simulink subsystem "FTC_Unknown"  (R2020b)
settings: Solver=VariableStepAuto  StartTime=0.0  StopTime=10.0  RelTol=1e-3
values from neighbouring files (symbols this model uses):
  B = [0.25   -1.4142/(4*l)     1.4142/(4*l)     1/(4*c) ... (first row only)    [H250_LOEUnknown_400HzParam.m]
  g = (9.8)    (= 9.8)    [H250_LOEKnown_400HzParam.m]    (also in H250_LOEUnknown_400HzParam.m; H333_LOEKnown_400HzParam.m)
  J = (diag([0.0056 0.0056 0.0104]))    [H250_LOEKnown_400HzParam.m]    (also in H250_LOEUnknown_400HzParam.m; H333_LOEKnown_400HzParam.m = (diag([0.012 0.0120 0.02])))
  m = (0.752)    (= 0.752)    [H250_LOEKnown_400HzParam.m]    (also in H250_LOEUnknown_400HzParam.m; H333_LOEKnown_400HzParam.m = 1.13)
  M = ([ 1          1          1         1 ... (first row only)    [H250_LOEKnown_400HzParam.m]    (also in H250_LOEUnknown_400HzParam.m; H333_LOEKnown_400HzParam.m)
  MY_ATT_P = Pixhawk_CSC.Parameter( {single(8), 'MY_ATT_P'}  )    [H250_LOEKnown_400HzParam.m]    (also in H250_LOEUnknown_400HzParam.m = Pixhawk_CSC.Parameter( {single(3), 'MY_ATT_P'}  ); H333_LOEKnown_400HzParam.m)
  MY_ATT_P_YAW = Pixhawk_CSC.Parameter( {single(0), 'MY_ATT_P_YAW'}  )    [H250_LOEKnown_400HzParam.m]    (also in H250_LOEUnknown_400HzParam.m = Pixhawk_CSC.Parameter( {single(0.0), 'MY_ATT_P_YAW'}  ); H333_LOEKnown_400HzParam.m)
  MY_POS_P = Pixhawk_CSC.Parameter( {single(0.5), 'MY_POS_P'}  )    [H250_LOEKnown_400HzParam.m]    (also in H250_LOEUnknown_400HzParam.m; H333_LOEKnown_400HzParam.m)
  MY_RATE_P = Pixhawk_CSC.Parameter( {single(12), 'MY_RATE_P'}  )    [H250_LOEKnown_400HzParam.m]    (also in H250_LOEUnknown_400HzParam.m = Pixhawk_CSC.Parameter( {single(14), 'MY_RATE_P'}  ); H333_LOEKnown_400HzParam.m)
  MY_RATE_P_YAW = Pixhawk_CSC.Parameter( {single(0.3), 'MY_RATE_P_YAW'}  )    [H250_LOEKnown_400HzParam.m]    (also in H250_LOEUnknown_400HzParam.m = Pixhawk_CSC.Parameter( {single(0.0), 'MY_RATE_P_YAW'}  ); H333_LOEKnown_400HzParam.m)
  MY_SAT_AD = Pixhawk_CSC.Parameter({single(0.13), 'MY_SAT_AD'} )    [H250_LOEKnown_400HzParam.m]    (also in H250_LOEUnknown_400HzParam.m; H333_LOEKnown_400HzParam.m)
  MY_TAU_P_A = Pixhawk_CSC.Parameter( {single(0), 'MY_TAU_P_A'}  )    [H250_LOEKnown_400HzParam.m]    (also in H250_LOEUnknown_400HzParam.m = Pixhawk_CSC.Parameter( {single(0.0), 'MY_TAU_P_A'}  ); H333_LOEKnown_400HzParam.m)
  MY_TAU_P_A_YAW = Pixhawk_CSC.Parameter( {single(0), 'MY_TAU_P_A_YAW'}  )    [H250_LOEKnown_400HzParam.m]    (also in H250_LOEUnknown_400HzParam.m; H333_LOEKnown_400HzParam.m)
  MY_TAU_P_P = Pixhawk_CSC.Parameter( {single(1.5), 'MY_TAU_P_P'}  )    [H250_LOEKnown_400HzParam.m]    (also in H250_LOEUnknown_400HzParam.m = Pixhawk_CSC.Parameter( {single(1.3), 'MY_TAU_P_P'}  ); H333_LOEKnown_400HzParam.m)
  MY_TAU_P_P_YAW = Pixhawk_CSC.Parameter( {single(0.1), 'MY_TAU_P_P_YAW'}  )    [H250_LOEKnown_400HzParam.m]    (also in H250_LOEUnknown_400HzParam.m; H333_LOEKnown_400HzParam.m)
  MY_VEL_P = Pixhawk_CSC.Parameter( {single(0.8), 'MY_VEL_P'}  )    [H250_LOEKnown_400HzParam.m]    (also in H250_LOEUnknown_400HzParam.m; H333_LOEKnown_400HzParam.m)
  T00 = single([m*g/4 m*g/4 m*g/4 m*g/4]')    [H250_LOEKnown_400HzParam.m]    (also in H250_LOEUnknown_400HzParam.m; H333_LOEKnown_400HzParam.m)
  Tf = 0.06    [H250_LOEKnown_400HzParam.m]    (also in H250_LOEUnknown_400HzParam.m; H333_LOEKnown_400HzParam.m)
  Tmotorbar = (0.035)    (= 0.035)    [H250_LOEKnown_400HzParam.m]    (also in H250_LOEUnknown_400HzParam.m = 0.032; H333_LOEKnown_400HzParam.m)
  Ts = 1/400    (= 0.0025)    [H250_LOEKnown_400HzParam.m]    (also in H250_LOEUnknown_400HzParam.m; H333_LOEKnown_400HzParam.m)
libraries: discretizing x10, simulink x1, sharedtransform x1, pid_lib x1, pixhawk_slib_uORB_RW x1
settings Model: Creator=kcx06  LastModifiedBy=kcx06

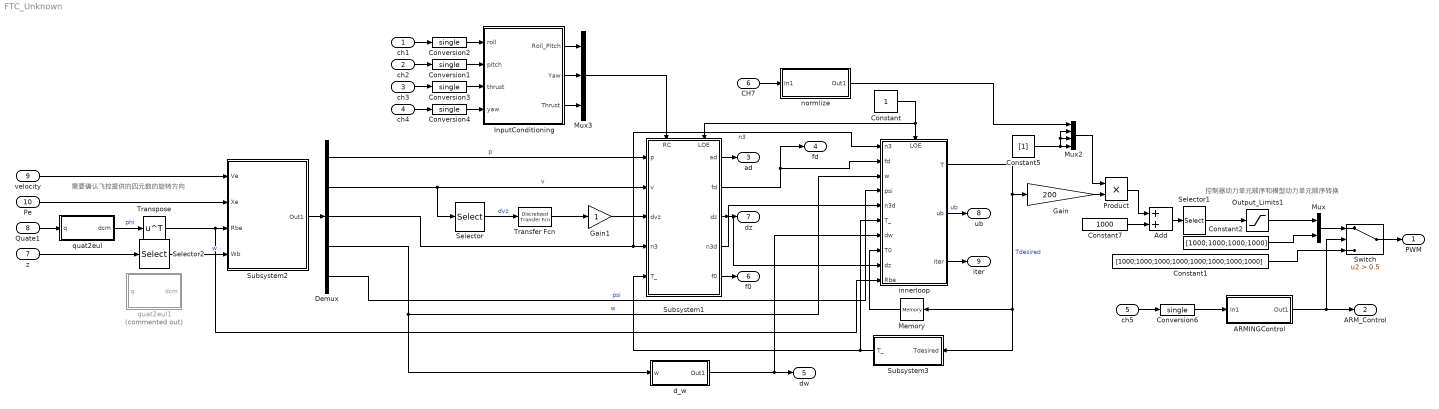
== system FTC_Unknown ==
  note: 需要确认飞控提供的四元数的旋转方向
  note: 控制器动力单元顺序和模型动力单元顺序转换
  ch1 : Inport  OutDataTypeStr=uint16  PortDimensions=1
  ch2 : Inport  Port=2  OutDataTypeStr=uint16  PortDimensions=1
  ch3 : Inport  Port=3  OutDataTypeStr=uint16  PortDimensions=1
  ch4 : Inport  Port=4  OutDataTypeStr=uint16  PortDimensions=1
  ch5 : Inport  Port=5  OutDataTypeStr=uint16  PortDimensions=1  Interpolate=off
  CH7 : Inport  Port=6
  z : Inport  Port=7
  Quate1 : Inport  Port=8
  velocity : Inport  Port=9
  Pe : Inport  Port=10
  ARMINGControl : Subsystem
  Add : Sum
  Constant : Constant  OutDataTypeStr=single
  Constant1 : Constant  Value=[1000;1000;1000;1000;1000;1000;1000;1000]  OutDataTypeStr=single
  Constant2 : Constant  Value=[1000;1000;1000;1000]  OutDataTypeStr=single
  Constant5 : Constant  Value=[1]  OutDataTypeStr=single
  Constant7 : Constant  Value=1000  OutDataTypeStr=single
  Conversion{1..4,6} (5 alike) : DataTypeConversion  OutDataTypeStr=single
  Demux : Demux  Outputs=[3 3 3 3 1]
  Gain : Gain  Gain=200
  Gain1 : Gain
  InputConditioning : Subsystem
  Memory : Memory  InitialCondition=T00
  Mux : Mux  Inputs=2
  Mux2 : Mux
  Mux3 : Mux  Inputs=3
  Output_Limits1 : Saturate  UpperLimit=2000  LowerLimit=1000
  Product : Product
  Selector : Selector  IndexMode=Zero-based  InputPortWidth=3  IndexOptions=Index vector (dialog)  Indices=[2]  OutputSizes=1
  Selector1 : Selector  IndexMode=Zero-based  InputPortWidth=4  IndexOptions=Index vector (dialog)  Indices=[0 2 3 1]  OutputSizes=1
  Selector2 : Selector  IndexMode=Zero-based  InputPortWidth=3  IndexOptions=Index vector (dialog)  Indices=[0 1 2]  OutputSizes=1
  Subsystem1 : Subsystem
      settings: PortSchema="{\"entries\":[{\"content\":{\"sides\":[{\"content\":{\"connectorIds\":[\"In1\",\"In2\",\"In3\",\"In4\",\"In5\"]},\"type\":\"ConnectorPlacement.EquallySpacedRectSide\",\"uuid\":\"59983f3e-2daf-41bd-bc3f-074c85f4b2eb\"},{\"content\":{\"connectorIds\":[\"Out1\",\"Out2\",\"Out3\",\"Out4\",\"Out5\"],\"side\":\"RIGHT\"},\"type\":\"ConnectorPlacement.EquallySpacedRectSide\",\"uuid\":\"6ee11e40-7870-4737-b9e6-fd7c25119100\"},{\"content\":{\"connectorIds\":[\"In6\",\"In7\"],\"side\":\"TOP\"},\"type\":\"ConnectorPlacement.EquallySpacedRectSide\",\"uuid\":\"847e9a02-4621-4cf8-a675-1479afa28be0\"}]},\"type\":\"ConnectorPlacement.EquallySpacedConnector\",\"uuid\":\"28981c41-e87e-4da3-ac2d-04a56d75ff2b\"}],\"packageUris\":[\"http://schema.mathworks.com/mf0/Connector/19700101\"],\"version\":\"1.0\"}"
  Subsystem2 : Subsystem
  Subsystem3 : Subsystem
  Switch : Switch  Criteria=u2 > Threshold  Threshold=0.5
  Transfer Fcn : discretizing/Discretized Transfer Fcn  Numerator=[1 0]  Denominator=[Tf 1]  AbsTol=auto  SampleTime=Ts  method=zoh  Wc=1
      settings: SourceProductBaseCode=SL
  Transpose : Math  Operator=transpose  SaturateOnIntegerOverflow=on
  d_w : Subsystem
  innerloop : Subsystem
      settings: PortSchema="{\"entries\":[{\"content\":{\"sides\":[{\"content\":{\"connectorIds\":[\"In1\",\"In2\",\"In3\",\"In4\",\"In5\",\"In6\",\"In7\",\"In8\",\"In9\",\"In10\"]},\"type\":\"ConnectorPlacement.EquallySpacedRectSide\",\"uuid\":\"43c6e1bd-c98b-47b4-98da-f51fdffff433\"},{\"content\":{\"connectorIds\":[\"Out1\",\"Out2\",\"Out3\"],\"side\":\"RIGHT\"},\"type\":\"ConnectorPlacement.EquallySpacedRectSide\",\"uuid\":\"ac1c9532-9168-4bf4-8fed-08d3fdc16453\"},{\"content\":{\"connectorIds\":[\"In11\"],\"side\":\"TOP\"},\"type\":\"ConnectorPlacement.EquallySpacedRectSide\",\"uuid\":\"32774b13-030c-47c6-b846-fc6c0ce2dd6f\"}]},\"type\":\"ConnectorPlacement.EquallySpacedConnector\",\"uuid\":\"dd62421a-d766-429a-a161-5a0f77c5a7ba\"}],\"packageUris\":[\"http://schema.mathworks.com/mf0/Connector/19700101\"],\"version\":\"1.0\"}"
  normlize : Subsystem
  quat2eul : MATLAB Function  TreatAsAtomicUnit=on
  quat2eul1 : MATLAB Function  Commented=on  TreatAsAtomicUnit=on
  PWM : Outport  PortDimensions=8  VectorParamsAs1DForOutWhenUnconnected=off
  ARM_Control : Outport  Port=2  PortDimensions=1  VectorParamsAs1DForOutWhenUnconnected=off
  ad : Outport  Port=3
  fd : Outport  Port=4
  dw : Outport  Port=5
  f0 : Outport  Port=6
  dz : Outport  Port=7
  ub : Outport  Port=8
  iter : Outport  Port=9
  wires:
  CH7/1 -> normlize/1(In1)
  z/1 -> Selector2/1
  Add/1 -> Selector1/1
  Subsystem1/1(ad) -> ad/1
  InputConditioning/3(Thrust) -> Mux3/3
  velocity/1 -> Subsystem2/1(Ve)
  Conversion2/1 -> InputConditioning/1(roll)
  Transpose/1 -> Subsystem2/3(Rbe), innerloop/10(Rbe)
  Demux/3 -> Subsystem1/4(n3), innerloop/1(n3)  "n3"
  InputConditioning/1(Roll_Pitch) -> Mux3/1
  Selector/1 -> Transfer Fcn/1  "dvz"
  Subsystem1/3(dz) -> dz/1, innerloop/9(dz)
  Product/1 -> Add/1
  Constant/1 -> innerloop/11(LOE), Subsystem1/7(LOE)
  Constant1/1 -> Switch/3
  Subsystem3/1(T_) -> Subsystem1/5(T_), innerloop/6(T_)
  quat2eul/1(dcm) -> Transpose/1  "phi"
  Demux/1 -> Subsystem1/1(p)  "p"
  Selector2/1 -> Subsystem2/4(Wb)  "w"
  innerloop/3(iter) -> iter/1
  Conversion3/1 -> InputConditioning/3(thrust)
  Pe/1 -> Subsystem2/2(Xe)
  ch5/1 -> Conversion6/1
  d_w/1(Out1) -> dw/1, innerloop/7(dw)
  Quate1/1 -> quat2eul/1(q)
  Demux/2 -> Subsystem1/2(v), Selector/1  "v"
  ch4/1 -> Conversion4/1
  Output_Limits1/1 -> Mux/1
  Constant7/1 -> Add/2
  Gain/1 -> Product/2
  Demux/4 -> innerloop/3(w), d_w/1(w)  "w"
  Subsystem1/2(fd) -> innerloop/2(fd), fd/1
  Memory/1 -> innerloop/8(T0)
  Demux/5 -> innerloop/4(psi)  "psi"
  ch1/1 -> Conversion2/1
  InputConditioning/2(Yaw) -> Mux3/2
  Selector1/1 -> Output_Limits1/1
  Transfer Fcn/1 -> Gain1/1
  innerloop/1(T) -> Gain/1, Memory/1, Subsystem3/1(Tdesired)  "Tdesired"
  ch2/1 -> Conversion1/1
  Conversion4/1 -> InputConditioning/4(yaw)
  normlize/1(Out1) -> Mux2/1
  Mux2/1 -> Product/1
  Mux/1 -> Switch/1
  Subsystem2/1(Out1) -> Demux/1
  innerloop/2(ub) -> ub/1  "ub"
  Conversion6/1 -> ARMINGControl/1(In1)
  Constant5/1 -> Mux2/4, Mux2/2, Mux2/3
  Switch/1 -> PWM/1
  Gain1/1 -> Subsystem1/3(dvz)
  ch3/1 -> Conversion3/1
  ARMINGControl/1(Out1) -> ARM_Control/1, Switch/2
  Subsystem1/5(f0) -> f0/1
  Mux3/1 -> Subsystem1/6(RC)
  Constant2/1 -> Mux/2
  Conversion1/1 -> InputConditioning/2(pitch)
  Subsystem1/4(n3d) -> innerloop/5(n3d)

== system FTC_Unknown/ARMINGControl ==
  In1 : Inport
  Compare To Constant3 : simulink/Logic and Bit Operations/Compare To Constant  relop=>=  const=uint16(1500)  OutDataTypeStr=boolean
  Out1 : Outport  VectorParamsAs1DForOutWhenUnconnected=off
  wires:
  In1/1 -> Compare To Constant3/1
  Compare To Constant3/1 -> Out1/1

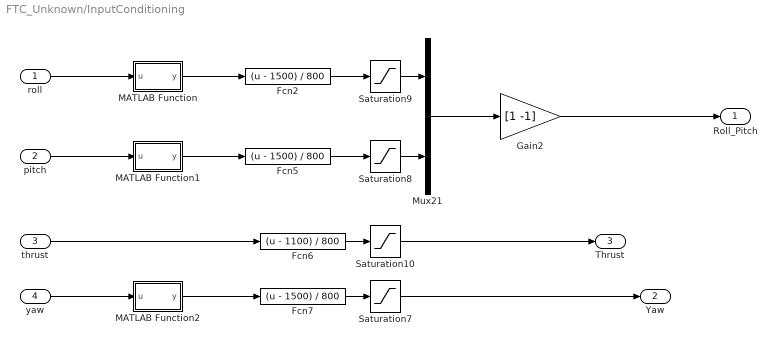
== system FTC_Unknown/InputConditioning ==
  roll : Inport
  pitch : Inport  Port=2
  thrust : Inport  Port=3
  yaw : Inport  Port=4
  Fcn2 : Fcn  Expr=(u - 1500) / 800
  Fcn5 : Fcn  Expr=(u - 1500) / 800
  Fcn6 : Fcn  Expr=(u - 1100) / 800
  Fcn7 : Fcn  Expr=(u - 1500) / 800
  Gain2 : Gain  Gain=[1 -1]  OutDataTypeStr=Inherit: Inherit via back propagation
  MATLAB Function : MATLAB Function  TreatAsAtomicUnit=on
  MATLAB Function1 : MATLAB Function  TreatAsAtomicUnit=on
  MATLAB Function2 : MATLAB Function  TreatAsAtomicUnit=on
  Mux21 : Mux  Inputs=2
  Saturation10 : Saturate  UpperLimit=1  LowerLimit=0
  Saturation7 : Saturate  UpperLimit=1  LowerLimit=-1
  Saturation8 : Saturate  UpperLimit=1  LowerLimit=-1
  Saturation9 : Saturate  UpperLimit=1  LowerLimit=-1
  Roll_Pitch : Outport  VectorParamsAs1DForOutWhenUnconnected=off
  Yaw : Outport  Port=2  VectorParamsAs1DForOutWhenUnconnected=off
  Thrust : Outport  Port=3  VectorParamsAs1DForOutWhenUnconnected=off
  wires:
  yaw/1 -> MATLAB Function2/1(u)
  MATLAB Function/1(y) -> Fcn2/1
  MATLAB Function1/1(y) -> Fcn5/1
  roll/1 -> MATLAB Function/1(u)
  thrust/1 -> Fcn6/1
  MATLAB Function2/1(y) -> Fcn7/1
  pitch/1 -> MATLAB Function1/1(u)
  Fcn7/1 -> Saturation7/1
  Saturation9/1 -> Mux21/1
  Fcn5/1 -> Saturation8/1
  Fcn2/1 -> Saturation9/1
  Fcn6/1 -> Saturation10/1
  Saturation8/1 -> Mux21/2
  Mux21/1 -> Gain2/1
  Gain2/1 -> Roll_Pitch/1
  Saturation7/1 -> Yaw/1
  Saturation10/1 -> Thrust/1

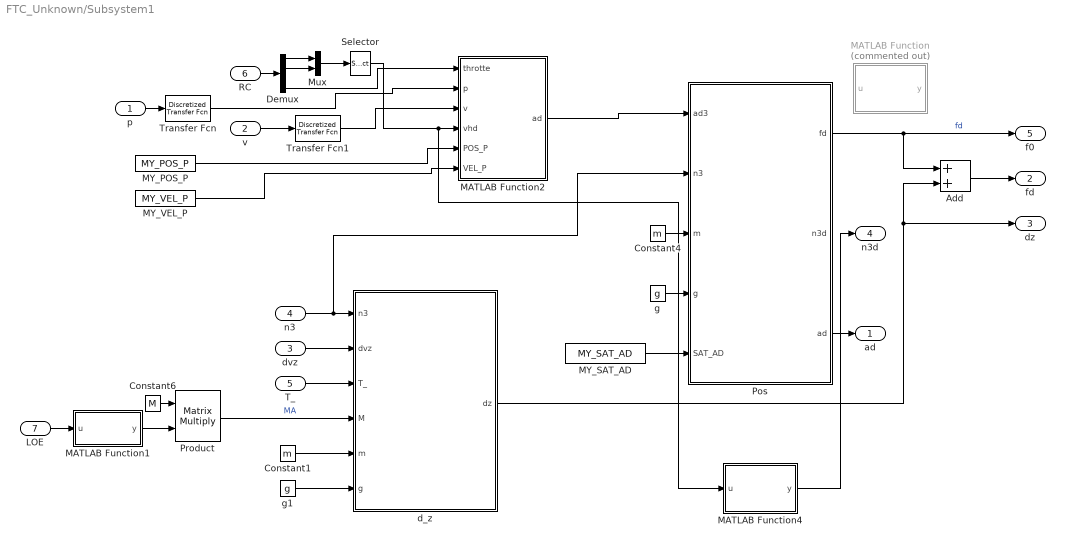
== system FTC_Unknown/Subsystem1 ==
  p : Inport
  v : Inport  Port=2
  dvz : Inport  Port=3
  n3 : Inport  Port=4
  T_ : Inport  Port=5
  RC : Inport  Port=6
  LOE : Inport  Port=7
  Add : Sum
  Constant1 : Constant  Value=m  OutDataTypeStr=single
  Constant4 : Constant  Value=m  OutDataTypeStr=single
  Constant6 : Constant  Value=M  OutDataTypeStr=single
  Demux : Demux
  MATLAB Function : MATLAB Function  Commented=on  TreatAsAtomicUnit=on
  MATLAB Function1 : MATLAB Function  TreatAsAtomicUnit=on
  MATLAB Function2 : MATLAB Function  TreatAsAtomicUnit=on
  MATLAB Function4 : MATLAB Function  TreatAsAtomicUnit=on
  MY_POS_P : Constant  Value=MY_POS_P
  MY_SAT_AD : Constant  Value=MY_SAT_AD
      settings: AttributesFormatString=|
      | 0.13
      | Default
  MY_VEL_P : Constant  Value=MY_VEL_P
  Mux : Mux  Inputs=2
  Pos : MATLAB Function  TreatAsAtomicUnit=on
  Product : Product  Multiplication=Matrix(*)
  Selector : Selector  IndexMode=Zero-based  InputPortWidth=2  IndexOptions=Index vector (dialog)  Indices=[1 0]  OutputSizes=1
  Transfer Fcn : discretizing/Discretized Transfer Fcn  Numerator=[1 ]  Denominator=[Tf 1]  AbsTol=auto  SampleTime=Ts  method=zoh  Wc=1
      settings: SourceProductBaseCode=SL
  Transfer Fcn1 : discretizing/Discretized Transfer Fcn  Numerator=[1 ]  Denominator=[Tf 1]  AbsTol=auto  SampleTime=Ts  method=zoh  Wc=1
      settings: SourceProductBaseCode=SL
  d_z : MATLAB Function  TreatAsAtomicUnit=on
  g : Constant  Value=g  OutDataTypeStr=single
  g1 : Constant  Value=g  OutDataTypeStr=single
  ad : Outport
  fd : Outport  Port=2
  dz : Outport  Port=3
  n3d : Outport  Port=4
  f0 : Outport  Port=5
  wires:
  MATLAB Function4/1(y) -> n3d/1
  MY_SAT_AD/1 -> Pos/5(SAT_AD)
  MY_VEL_P/1 -> MATLAB Function2/6(VEL_P)
  MY_POS_P/1 -> MATLAB Function2/5(POS_P)
  Selector/1 -> MATLAB Function2/4(vhd), MATLAB Function4/1(u)
  Mux/1 -> Selector/1
  Demux/2 -> Mux/2
  Demux/1 -> Mux/1
  Transfer Fcn1/1 -> MATLAB Function2/3(v)
  MATLAB Function2/1(ad) -> Pos/1(ad3)
  Demux/4 -> MATLAB Function2/1(throtte)
  RC/1 -> Demux/1
  Product/1 -> d_z/4(M)  "MA"
  Constant6/1 -> Product/1
  LOE/1 -> MATLAB Function1/1(u)
  MATLAB Function1/1(y) -> Product/2
  n3/1 -> d_z/1(n3), Pos/2(n3)
  Transfer Fcn/1 -> MATLAB Function2/2(p)
  d_z/1(dz) -> Add/2, dz/1
  Add/1 -> fd/1
  g1/1 -> d_z/6(g)
  Constant1/1 -> d_z/5(m)
  g/1 -> Pos/4(g)
  Constant4/1 -> Pos/3(m)
  v/1 -> Transfer Fcn1/1
  T_/1 -> d_z/3(T_)
  p/1 -> Transfer Fcn/1
  Pos/1(fd) -> Add/1, f0/1  "fd"
  dvz/1 -> d_z/2(dvz)
  Pos/3(ad) -> ad/1

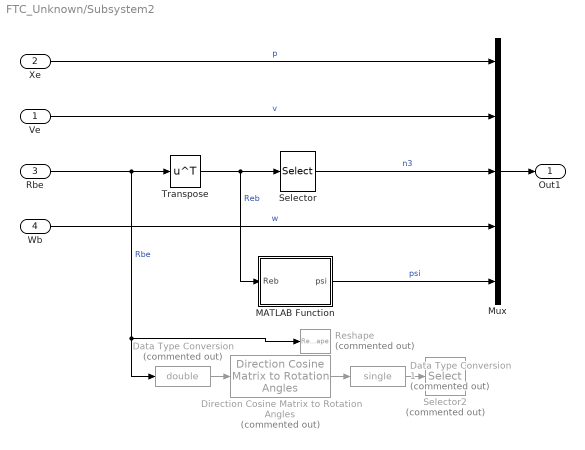
== system FTC_Unknown/Subsystem2 ==
  Ve : Inport
  Xe : Inport  Port=2
  Rbe : Inport  Port=3
  Wb : Inport  Port=4
  Data Type Conversion : DataTypeConversion  Commented=on  OutDataTypeStr=double
  Data Type Conversion1 : DataTypeConversion  Commented=on  OutDataTypeStr=single
  Direction Cosine Matrix to Rotation Angles : sharedtransform/Direction Cosine Matrix to Rotation Angles  Commented=on  rotationOrder=ZYX  aMode=aMode  action=None  tolerance=eps(2)
      settings: SourceProductBaseCode=AE,PW,MT,UV,VE,VP
  MATLAB Function : MATLAB Function  TreatAsAtomicUnit=on
  Mux : Mux  Inputs=[3 3 3 3 1]
  Reshape : Reshape  Commented=on
  Selector : Selector  NumberOfDimensions=2  IndexMode=Zero-based  InputPortWidth=3  IndexOptions=Select all,Index vector (dialog)  Indices=[1 3],2  OutputSizes=1,1
  Selector2 : Selector  Commented=on  InputPortWidth=3  IndexOptions=Index vector (dialog)  Indices=[3 2 1]  OutputSizes=1
  Transpose : Math  Operator=transpose  SaturateOnIntegerOverflow=on
  Out1 : Outport
  wires:
  Data Type Conversion1/1 -> Selector2/1
  Data Type Conversion/1 -> Direction Cosine Matrix to Rotation Angles/1
  Direction Cosine Matrix to Rotation Angles/1 -> Data Type Conversion1/1
  MATLAB Function/1(psi) -> Mux/5  "psi"
  Wb/1 -> Mux/4  "w"
  Mux/1 -> Out1/1
  Selector/1 -> Mux/3  "n3"
  Transpose/1 -> Selector/1, MATLAB Function/1(Reb)  "Reb"
  Rbe/1 -> Transpose/1, Data Type Conversion/1, Reshape/1  "Rbe"
  Ve/1 -> Mux/2  "v"
  Xe/1 -> Mux/1  "p"

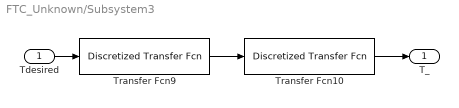
== system FTC_Unknown/Subsystem3 ==
  Tdesired : Inport
  Transfer Fcn10 : discretizing/Discretized Transfer Fcn  Numerator=[1]  Denominator=[Tmotorbar 1]  AbsTol=auto  SampleTime=Ts  method=zoh  Wc=1
      settings: SourceProductBaseCode=SL
  Transfer Fcn9 : discretizing/Discretized Transfer Fcn  Numerator=[1]  Denominator=[Tf 1]  AbsTol=auto  SampleTime=Ts  method=zoh  Wc=1
      settings: SourceProductBaseCode=SL
  T_ : Outport
  wires:
  Transfer Fcn9/1 -> Transfer Fcn10/1
  Tdesired/1 -> Transfer Fcn9/1
  Transfer Fcn10/1 -> T_/1

== system FTC_Unknown/d_w ==
  w : Inport
  Transfer Fcn4 : discretizing/Discretized Transfer Fcn  Numerator=[1 0]  Denominator=[Tf 1]  AbsTol=auto  SampleTime=Ts  method=zoh  Wc=1
      settings: SourceProductBaseCode=SL
  Out1 : Outport
  wires:
  Transfer Fcn4/1 -> Out1/1
  w/1 -> Transfer Fcn4/1

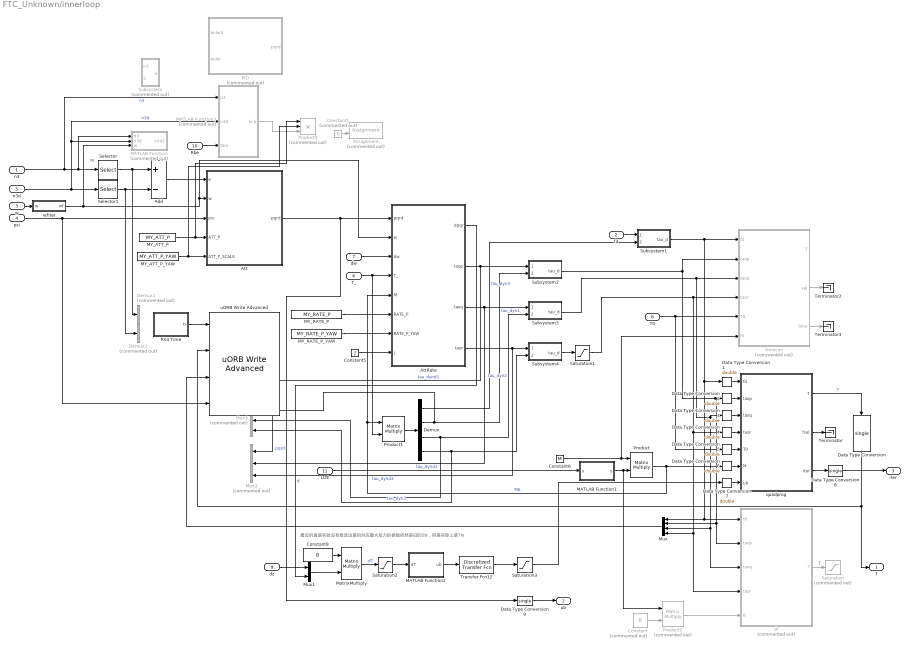
== system FTC_Unknown/innerloop ==
  note: 最近的真是实验没有修改这里的对应最大拉力的参数依然是旧的5N，但是实际上是7N
  note: PI
  n3 : Inport
  fd : Inport  Port=2
  w : Inport  Port=3
  psi : Inport  Port=4
  n3d : Inport  Port=5
  T_ : Inport  Port=6
  dw : Inport  Port=7
  T0 : Inport  Port=8
  dz : Inport  Port=9
  Rbe : Inport  Port=10
  LOE : Inport  Port=11
  Add : Sum  Inputs=+-
  Assignment : Assignment  Commented=on  DiagnosticForDimensions=Warning  IndexOptions=Index vector (dialog)  Indices=3  OutputSizes=1
  Att : MATLAB Function  TreatAsAtomicUnit=on
  AttRate : MATLAB Function  TreatAsAtomicUnit=on
  Constant : Constant  Commented=on  Value=B  OutDataTypeStr=single
  Constant1 : Constant  Commented=on  Value=0  OutDataTypeStr=single
  Constant5 : Constant  Value=J  OutDataTypeStr=single
  Constant6 : Constant  Value=M  OutDataTypeStr=single
  Constant8 : Constant  Value=B
  Data Type Conversion : DataTypeConversion  OutDataTypeStr=single
  Data Type Conversion{1..7} (7 alike) : DataTypeConversion  OutDataTypeStr=double
  Data Type Conversion8 : DataTypeConversion  OutDataTypeStr=single
  Data Type Conversion9 : DataTypeConversion  OutDataTypeStr=single
  Demux : Demux
  Demux1 : Demux  Commented=on  Outputs=2
  Demux2 : Demux  Commented=on  Outputs=2
  MATLAB Function : MATLAB Function  Commented=on  TreatAsAtomicUnit=on
  MATLAB Function1 : MATLAB Function  TreatAsAtomicUnit=on
  MATLAB Function2 : MATLAB Function  TreatAsAtomicUnit=on
  MATLAB Function3 : MATLAB Function  Commented=on  TreatAsAtomicUnit=on
  MY_ATT_P : Constant  Value=MY_ATT_P
  MY_ATT_P_YAW : Constant  Value=MY_ATT_P_YAW
  MY_RATE_P : Constant  Value=MY_RATE_P
  MY_RATE_P_YAW : Constant  Value=MY_RATE_P_YAW
  MatrixMultiply : Product  Multiplication=Matrix(*)
  Mux : Mux
  Mux1 : Mux  Inputs=2
  Mux2 : Mux  Commented=on  Inputs=3
  Mux3 : Mux  Commented=on  Inputs=3
  PID : MATLAB Function  Commented=on  TreatAsAtomicUnit=on
  PX4 Time : MATLAB Function  TreatAsAtomicUnit=on
  Product : Product  Multiplication=Matrix(*)
  Product1 : Product  Multiplication=Matrix(*)
  Product2 : Product  Commented=on  Multiplication=Matrix(*)
  Product3 : Product  Commented=on  Inputs=3
  Saturation : Saturate  Commented=on  UpperLimit=[3 3 3 3]  LowerLimit=[0 0 0 0]  OutDataTypeStr=single
  Saturation1 : Saturate  UpperLimit=0.075  LowerLimit=-0.075
  Saturation2 : Saturate  UpperLimit=5  LowerLimit=-5
  Saturation3 : Saturate  UpperLimit=5  LowerLimit=0
  Selector : Selector  IndexMode=Zero-based  InputPortWidth=3  IndexOptions=Index vector (dialog)  Indices=[0 1]  OutputSizes=1
  Selector1 : Selector  IndexMode=Zero-based  InputPortWidth=3  IndexOptions=Index vector (dialog)  Indices=[0 1]  OutputSizes=1
  Subsystem : Subsystem  Commented=on
  Subsystem1 : Subsystem
  Subsystem2 : Subsystem
  Subsystem3 : Subsystem
  Subsystem4 : Subsystem
  Terminator : Terminator
  Terminator2 : Terminator
  Terminator3 : Terminator
  Transfer Fcn12 : discretizing/Discretized Transfer Fcn  Numerator=[1]  Denominator="[1.7  1]"  AbsTol=auto  SampleTime=Ts  method=zoh  Wc=40
      link override Discrete Transfer Fcn: InitialStates=[5;5;5;5]
      settings: SourceProductBaseCode=SL
  dr : MATLAB Function  Commented=on  TreatAsAtomicUnit=on
  fmincon : MATLAB Function  Commented=on  TreatAsAtomicUnit=on
  quadprog : MATLAB Function  TreatAsAtomicUnit=on
  uORB Write Advanced : pixhawk_slib_uORB_RW/uORB Write Advanced  Ts=0  uORB_AdvtQueue=on  uORB_FieldEnabledArr="0  0  0  1  0  0  0  0  0  0  0"  uORB_Topic_str=0  uORB_Struct_DT="[1  1  1  1  1]"  BlockInputCount=5  uORB_StructParams="[\"voltage_v\",\"voltage_filtered_v\",\"current_a\",\"current_filtered_a\",\"remaining\"]"  uORB_PortSizes="[1  1  1  1]"  MsgSizeOf=0  MW_update=true
      settings: SourceProductName=Pixhawk Target Blocks
  wfiter : Subsystem
  T : Outport  PortDimensions=4
  ub : Outport  Port=2
  iter : Outport  Port=3
  wires:
  Selector/1 -> Demux1/1, Add/1
  Selector1/1 -> Add/2, Demux2/1
  PX4 Time/1(ts) -> uORB Write Advanced/1
  Constant1/1 -> Assignment/2
  MATLAB Function3/1(ncb) -> Product3/3
  Rbe/1 -> MATLAB Function3/3(Rbe)
  Data Type Conversion9/1 -> ub/1
  Add/1 -> Att/1(e)
  Saturation3/1 -> Data Type Conversion7/1
  Transfer Fcn12/1 -> Saturation3/1
  MatrixMultiply/1 -> Saturation2/1  "dT"
  Saturation2/1 -> MATLAB Function2/1(dT)
  dz/1 -> Mux1/1
  Mux1/1 -> MatrixMultiply/2
  Constant8/1 -> MatrixMultiply/1
  MATLAB Function2/1(ub) -> Transfer Fcn12/1
  n3d/1 -> Selector1/1, MATLAB Function/2(n3d), MATLAB Function3/2(n3d)  "n3d"
  MY_ATT_P_YAW/1 -> Att/5(ATT_P_SCALE), Product3/2
  MY_ATT_P/1 -> Product3/1, Att/4(ATT_P)
  MY_RATE_P_YAW/1 -> AttRate/7(RATE_P_YAW)
  MY_RATE_P/1 -> AttRate/6(RATE_P)
  Data Type Conversion/1 -> uORB Write Advanced/2, T/1
  MATLAB Function1/1(y) -> Product/2, Product2/1
  Constant/1 -> Product2/2
  Att/1(pqrd) -> Data Type Conversion9/1, AttRate/1(pqrd)  "pqrd"
  Product1/1 -> Demux/1
  n3/1 -> MATLAB Function3/1(n3), MATLAB Function/1(n3), Selector/1  "n3"
  Product/1 -> Data Type Conversion6/1, AttRate/5(M), Product1/1  "MA"
  LOE/1 -> MATLAB Function1/1(u)
  Saturation1/1 -> fmincon/4(taor), Data Type Conversion4/1, dr/4(taor), Mux/4
  Demux/4 -> Subsystem4/2(tau_dyn), Mux3/3  "tau_dyn3"
  AttRate/4(taor) -> Mux2/3, Subsystem4/1(tau_dynd)  "tau_dynd3"
  Demux/3 -> Subsystem3/2(tau_dyn), Mux3/2  "tau_dyn2"
  AttRate/3(taoq) -> Mux2/2, Subsystem3/1(tau_dynd)  "tau_dynd2"
  Demux/2 -> Subsystem2/2(tau_dyn), Mux3/1  "tau_dyn1"
  AttRate/2(taop) -> Subsystem2/1(tau_dynd), Mux2/1  "tau_dynd1"
  fd/1 -> Subsystem1/1(tau_dynd)
  Demux/1 -> Subsystem1/2(tau_dyn)  "tau_dyn3"
  Data Type Conversion8/1 -> iter/1
  quadprog/3(iter) -> Data Type Conversion8/1
  Subsystem1/1(tau_d) -> fmincon/1(fd), Data Type Conversion1/1, dr/1(fd), Mux/1
  Subsystem4/1(tau_d) -> Saturation1/1
  Subsystem3/1(tau_d) -> fmincon/3(taoq), Data Type Conversion3/1, dr/3(taoq), Mux/3
  Subsystem2/1(tau_d) -> Data Type Conversion2/1, dr/2(taop), Mux/2, fmincon/2(taop)
  Data Type Conversion7/1 -> quadprog/7(ub)
  Data Type Conversion6/1 -> quadprog/6(M)
  Data Type Conversion5/1 -> quadprog/5(T0)
  Data Type Conversion4/1 -> quadprog/4(taor)
  Data Type Conversion3/1 -> quadprog/3(taoq)
  Data Type Conversion2/1 -> quadprog/2(taop)
  Data Type Conversion1/1 -> quadprog/1(fd)
  quadprog/1(T) -> Data Type Conversion/1  "T"
  wfiter/1(wf) -> AttRate/2(w), Att/2(w), MATLAB Function/3(w)
  w/1 -> wfiter/1(w)
  psi/1 -> uORB Write Advanced/4, Att/3(psi)
  Product2/1 -> dr/5(B)
  fmincon/3(time) -> Terminator3/1
  fmincon/2(val) -> Terminator2/1
  dr/1(T) -> Saturation/1  "T"
  quadprog/2(fval) -> Terminator/1
  Constant6/1 -> Product/1, fmincon/6(M)
  Constant5/1 -> AttRate/8(J)
  T_/1 -> AttRate/4(T_), Product1/2
  T0/1 -> Data Type Conversion5/1, fmincon/5(T0)
  AttRate/1(dpqr) -> Mux1/2  "d"
  dw/1 -> AttRate/3(dw)
  Mux/1 -> uORB Write Advanced/3

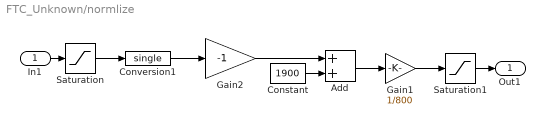
== system FTC_Unknown/normlize ==
  In1 : Inport
  Add : Sum
  Constant : Constant  Value=1900  OutDataTypeStr=single
  Conversion1 : DataTypeConversion  OutDataTypeStr=single
  Gain1 : Gain  Gain=1/800
  Gain2 : Gain  Gain=-1
  Saturation : Saturate  UpperLimit=1900  LowerLimit=1100
  Saturation1 : Saturate  UpperLimit=1  LowerLimit=0
  Out1 : Outport
  wires:
  Saturation1/1 -> Out1/1
  Conversion1/1 -> Gain2/1
  Constant/1 -> Add/2
  In1/1 -> Saturation/1
  Add/1 -> Gain1/1
  Gain1/1 -> Saturation1/1
  Gain2/1 -> Add/1
  Saturation/1 -> Conversion1/1

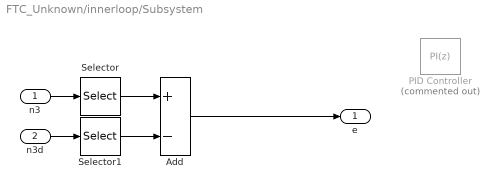
== system FTC_Unknown/innerloop/Subsystem ==
  n3 : Inport
  n3d : Inport  Port=2
  Add : Sum  Inputs=+-
  PID Controller : pid_lib/PID Controller  Commented=on  Controller=PI  Form=Parallel  TimeDomain=Discrete-time  UseExternalTs=off  SampleTime=-1  IntegratorMethod=Forward Euler  FilterMethod=Forward Euler  ControllerParametersSource=internal  P=0.8  I=0.05  D=0.02  UseFilter=on  N=100  TunerSelectOption=Transfer Function Based (PID Tuner App)  InitialConditionSource=internal  InitialConditionForIntegrator=0  InitialConditionForFilter=0  DifferentiatorICPrevScaledInput=0  ExternalReset=none  TrackingMode=off  Kt=1  LimitOutput=off  SatLimitsSource=internal  UpperSaturationLimit=0.3  LowerSaturationLimit=-0.3  LinearizeAsGain=on  AntiWindupMode=clamping  Kb=1  POutMin=[]  POutMax=[]  IOutMin=[]  IOutMax=[]  DOutMin=[]  DOutMax=[]  NOutMin=[]  NOutMax=[]  SumOutMin=[]  SumOutMax=[]  SaturationOutMin=[]  SaturationOutMax=[]  PParamMin=[]  PParamMax=[]  IParamMin=[]  IParamMax=[]  DParamMin=[]  DParamMax=[]  NParamMin=[]  NParamMax=[]  KbParamMin=[]  KbParamMax=[]  KtParamMin=[]  KtParamMax=[]  KbOutMin=[]  KbOutMax=[]  KtOutMin=[]  KtOutMax=[]  IntegratorOutMin=[]  IntegratorOutMax=[]  FilterOutMin=[]  FilterOutMax=[]  SumI1OutMin=[]  SumI1OutMax=[]  SumI2OutMin=[]  SumI2OutMax=[]  SumI3OutMin=[]  SumI3OutMax=[]  SumI4OutMin=[]  SumI4OutMax=[]  SumDOutMin=[]  SumDOutMax=[]  DifferentiatorOutMin=[]  DifferentiatorOutMax=[]  FilterDiffOutCoefMin=[]  FilterDiffOutCoefMax=[]  ReciprocalOutMin=[]  ReciprocalOutMax=[]  SumDenOutMin=[]  SumDenOutMax=[]  SumNumOutMin=[]  SumNumOutMax=[]  DivideOutMin=[]  DivideOutMax=[]  UdiffTsProdOutMin=[]  UdiffTsProdOutMax=[]  NTsProdOutMin=[]  NTsProdOutMax=[]  UintegralTsProdOutMin=[]  UintegralTsProdOutMax=[]  UngainTsProdOutMin=[]  UngainTsProdOutMax=[]  IntegratorContinuousStateAttributes=''  IntegratorStateMustResolveToSignalObject=off  IntegratorRTWStateStorageClass=Auto  FilterContinuousStateAttributes=''  FilterStateMustResolveToSignalObject=off  FilterRTWStateStorageClass=Auto  ParallelPVariant=InternalParameters  IdealPVariant=Disabled  IVariant=InternalParameters  DVariant=Disabled  IntegratorVariant=Discrete  SatVariant=Disabled  AWVariant=Passthrough  PCopyVariant=Disabled  TRVariant=Disabled  FdbkBlocksVariant=Forward  IdealPFdbkVariant=Disabled  SatFdbkVariant=Disabled  DerivativeFilterVariant=Disabled  NVariant=Disabled  NCopyVariant=Disabled_SignalSpec  FilterICVariant=Disabled  IntegratorICVariant=InternalICs  ExternalResetVariant=Disabled  TRSumVariant=Passthrough  SumFdbkVariant=Disabled  SumVariant=Sum_PI  TsampFilterVariant=InternalTs  TsampNgainVariant=Passthrough  TsampIntegralVariant=Passthrough  ExternalSaturationOutDataTypeStr=Inherit: Same as second input
  Selector : Selector  IndexMode=Zero-based  InputPortWidth=3  IndexOptions=Index vector (dialog)  Indices=[0 1]  OutputSizes=1
  Selector1 : Selector  IndexMode=Zero-based  InputPortWidth=3  IndexOptions=Index vector (dialog)  Indices=[0 1]  OutputSizes=1
  e : Outport
  wires:
  Add/1 -> e/1
  Selector1/1 -> Add/2
  Selector/1 -> Add/1
  n3d/1 -> Selector1/1
  n3/1 -> Selector/1

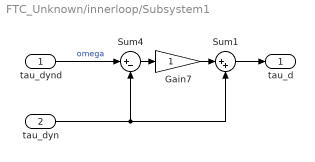
== system FTC_Unknown/innerloop/Subsystem1 ==
  tau_dynd : Inport
  tau_dyn : Inport  Port=2
  Gain7 : Gain
  Sum1 : Sum  Inputs=|++
  Sum4 : Sum  Inputs=|+-
  tau_d : Outport
  wires:
  tau_dyn/1 -> Sum4/2, Sum1/2
  Sum1/1 -> tau_d/1
  Sum4/1 -> Gain7/1
  Gain7/1 -> Sum1/1
  tau_dynd/1 -> Sum4/1  "omega"

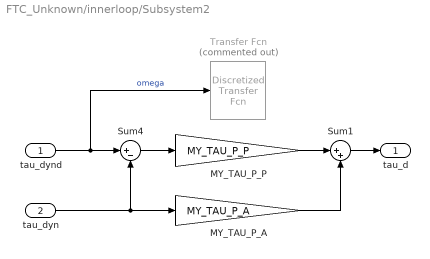
== system FTC_Unknown/innerloop/Subsystem2 ==
  tau_dynd : Inport
  tau_dyn : Inport  Port=2
  MY_TAU_P_A : Gain  Gain=MY_TAU_P_A
  MY_TAU_P_P : Gain  Gain=MY_TAU_P_P
  Sum1 : Sum  Inputs=|++
  Sum4 : Sum  Inputs=|+-
  Transfer Fcn : discretizing/Discretized Transfer Fcn  Commented=on  Numerator=[0.005 0]  Denominator=[Tf 1]  AbsTol=auto  SampleTime=Ts  method=zoh  Wc=1
      settings: SourceProductBaseCode=SL
  tau_d : Outport
  wires:
  MY_TAU_P_P/1 -> Sum1/1
  MY_TAU_P_A/1 -> Sum1/2
  tau_dynd/1 -> Sum4/1, Transfer Fcn/1  "omega"
  Sum4/1 -> MY_TAU_P_P/1
  Sum1/1 -> tau_d/1
  tau_dyn/1 -> MY_TAU_P_A/1, Sum4/2

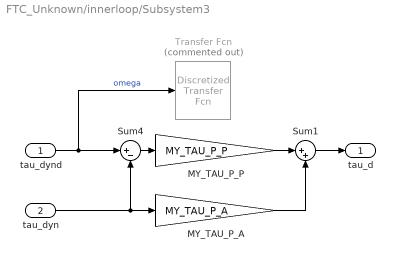
== system FTC_Unknown/innerloop/Subsystem3 ==
  tau_dynd : Inport
  tau_dyn : Inport  Port=2
  MY_TAU_P_A : Gain  Gain=MY_TAU_P_A
  MY_TAU_P_P : Gain  Gain=MY_TAU_P_P
  Sum1 : Sum  Inputs=|++
  Sum4 : Sum  Inputs=|+-
  Transfer Fcn : discretizing/Discretized Transfer Fcn  Commented=on  Numerator=[0.005 0]  Denominator=[Tf 1]  AbsTol=auto  SampleTime=Ts  method=zoh  Wc=1
      settings: SourceProductBaseCode=SL
  tau_d : Outport
  wires:
  MY_TAU_P_P/1 -> Sum1/1
  MY_TAU_P_A/1 -> Sum1/2
  tau_dyn/1 -> MY_TAU_P_A/1, Sum4/2
  Sum1/1 -> tau_d/1
  Sum4/1 -> MY_TAU_P_P/1
  tau_dynd/1 -> Sum4/1, Transfer Fcn/1  "omega"

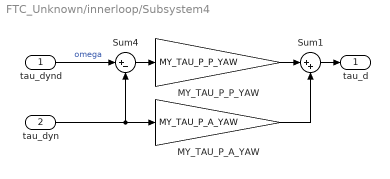
== system FTC_Unknown/innerloop/Subsystem4 ==
  tau_dynd : Inport
  tau_dyn : Inport  Port=2
  MY_TAU_P_A_YAW : Gain  Gain=MY_TAU_P_A_YAW
  MY_TAU_P_P_YAW : Gain  Gain=MY_TAU_P_P_YAW
  Sum1 : Sum  Inputs=|++
  Sum4 : Sum  Inputs=|+-
  tau_d : Outport
  wires:
  MY_TAU_P_A_YAW/1 -> Sum1/2
  tau_dynd/1 -> Sum4/1  "omega"
  MY_TAU_P_P_YAW/1 -> Sum1/1
  Sum4/1 -> MY_TAU_P_P_YAW/1
  Sum1/1 -> tau_d/1
  tau_dyn/1 -> Sum4/2, MY_TAU_P_A_YAW/1

== system FTC_Unknown/innerloop/wfiter ==
  w : Inport
  Transfer Fcn4 : discretizing/Discretized Transfer Fcn  Numerator=[1]  Denominator=[Tf 1]  AbsTol=auto  SampleTime=Ts  method=zoh  Wc=1
      settings: SourceProductBaseCode=SL
  wf : Outport
  wires:
  w/1 -> Transfer Fcn4/1
  Transfer Fcn4/1 -> wf/1

== matlab function FTC_Unknown/Subsystem1/MATLAB Function ==
  data: u input; y output
function y = fcn(u)
if u<0.9
y = single(0);
else
y = single(1);
end

== matlab function FTC_Unknown/Subsystem1/MATLAB Function1 ==
  data: u input; y output
function y = fcn(u)
y=diag([u,1,1,1]);

== matlab function FTC_Unknown/quat2eul1 ==
  data: q input single; dcm output single
function dcm  = quat2eul(q)
% Conversion from Quaternion to Euler angles based on the PX4 Firmware
% v1.6.5 release.
% 
% Quaternion -> DCM -> Euler Angles
% INPUT:
%   q: Quaternion vector of the format: (a + bi + cj + dk)
% OUTPUT:
%   [phi,theta,psi]: Euler angles in radians.
% 
 if norm(q)~=0
    a = q(1);
    b = q(2);
    c = q(3);
    d = q(4);

    aSq = a*a;
    bSq = b*b;
    cSq = c*c;
    dSq = d*d;

    d_pi2 = pi/2;

    % quaternion_to_dcm
    dcm00 = aSq + bSq - cSq - dSq;
    dcm01 = 2*(b*c - a*d);
    dcm02 = 2*(a*c + b*d);
    dcm10 = 2*(b*c + a*d);
    dcm11 = aSq - bSq + cSq - dSq;
    dcm12 = 2*(c*d - a*b);
    dcm20 = 2*(b*d - a*c);
    dcm21 = 2*(a*b + c*d);
    dcm22 = aSq - bSq - cSq + dSq;
    dcm=[dcm00 dcm01 dcm02;
              dcm10 dcm11 dcm12;
              dcm20 dcm21  dcm22];
 else
     dcm = single(eye(3,3));
 end
    % dcm_to_euler

== matlab function FTC_Unknown/innerloop/MATLAB Function ==
  data: n3 input; n3d2 output; n3d input; w input
function n3d2 = fcn(n3, n3d, w)
if abs(w(3))>pi
    % costheta   = dot(n3, n3d);
    costhetaXY = dot([n3(1:2);0], [n3d(1:2);0])/(norm([n3(1:2);0])*norm([n3d(1:2);0]));
    % sintheta   = cross(n3, n3d);
    sinthetaXY = cross([n3(1:2);0], [n3d(1:2);0])/(norm([n3(1:2);0])*norm([n3d(1:2);0]));

%     if sinthetaXY(3) > 0  
        %俯视下顺时针，与1号电机停止后机体旋转方向相反，不符合陀螺进动方向      
    %% s1 没有测试（预计没有明显改善）   
    %     n3d = [-n3d(1)/1; -n3d(2)/1; n3d(3)];
    %% s2 位置超调略大
    %     n3d = [single(0); single(0); single(1.0)];
    %% s3 位置超调过大
    %     n3d = [-n3(1)/3; -n3(2)/3; n3(3)];
    %     n3d = n3d/norm(n3d); 
%     end


    %% s4
    % if costhetaXY <0.9397  %只考虑夹角大小不管转向是否符合陀螺进动方向,大于20°满足
    %     n3d = [single(0); single(0); single(1.0)];
    % end

    %% s5
    if costhetaXY <0.8660 && sinthetaXY(3) > 0 %考虑夹角大小和是否符合陀螺进动方向大于20°满足
        n3d = [single(0); single(0); single(1.0)];
    end

    %% s6
    % if costheta <0.9397  %只考虑夹角大小不管转向是否符合陀螺进动方向,大于20°满足
    %     n3d = [single(0); single(0); single(1.0)];
    % end

    %% s7
    % if costheta <0.9397 && sinthetaXY(3) > 0 %考虑夹角大小和是否符合陀螺进动方向大于20°满足
    %     n3d = [single(0); single(0); single(1.0)];
    % end
end
n3d2 = n3d;

== matlab function FTC_Unknown/innerloop/PID ==
  data: eulerd input; euler input; pqrd output
function pqrd  = fcn(eulerd, euler)
k1 = 3;
pqd = k1 * [eulerd(1)-euler(1);eulerd(2)-euler(2)];
pqrd = [pqd;0];

== matlab function FTC_Unknown/innerloop/MATLAB Function3 ==
  data: n3 input; ncb output; n3d input; Rbe input
function ncb = fcn(n3, n3d, Rbe)
nc = cross(n3, n3d);
ncb  = Rbe*nc;

== matlab function FTC_Unknown/Subsystem1/MATLAB Function4 ==
  data: u input; y output
function y = fcn(u)
y = [-u/4; 1]/norm([-u/4; 1]);

== matlab function FTC_Unknown/innerloop/PX4 Time ==
  data: ts output
function ts  = fcn
% coder.cinclude('drivers/drv_hrt.h');
persistent count
if isempty(count)
    count = 0;
end

hrt = 0;
if coder.target('Rtw')
    hrt = coder.ceval('hrt_absolute_time');
else
    hrt = count;
end
ts = hrt;% us

count = count + 1;

== matlab function FTC_Unknown/innerloop/AttRate ==
  data: pqrd input; w input; dw input; T_ input; M input; RATE_P input; RATE_P_YAW input; J input; dpqr output size=3; taop output; taoq output; taor output
function [dpqr, taop, taoq, taor] = fcn(pqrd, w, dw, T_, M, RATE_P, RATE_P_YAW, J)
pqd = pqrd(1:2);
rd    = pqrd(3);
%% 角速率控制器计算

k2 = RATE_P;
k2_scaled = k2*RATE_P_YAW;

% kr = 0.001;
% dp =  M(2,:)*T_ - J(1,1)*dw(1) - kr*abs(w(1))*w(1) + w(2)*w(3)*(J(2,2)-J(3,3));
% dq =  M(3,:)*T_ - J(2,2)*dw(2) - kr*abs(w(2))*w(2) + w(3)*w(1)*(J(3,3)-J(1,1));
% dr  =  M(4,:)*T_ - J(3,3)*dw(3) - kr*abs(w(3))*w(3) + w(1)*w(2)*(J(1,1)-J(2,2));
dp = M(2,:)*T_ -J(1,1)*dw(1);
dq = M(3,:)*T_ -J(2,2)*dw(2);
dr  = M(4,:)*T_ -J(3,3)*dw(3);

% taop =            J(1,1)*k2*(pqd(1)-w(1)) + kr*abs(w(1))*w(1) - w(2)*w(3)*(J(2,2)-J(3,3))+dp;
% taoq =            J(2,2)*k2*(pqd(2)-w(2)) + kr*abs(w(2))*w(2) - w(3)*w(1)*(J(3,3)-J(1,1))+dq;
% taor  = mysatsingle(J(3,3)*k2_scaled*(rd-w(3)) + kr*abs(w(3))*w(3) - w(1)*w(2)*(J(1,1)-J(2,2))+dr,10.0);
taop =           J(1,1)*k2*(pqd(1)-w(1))+1.0*dp;
taoq =           J(2,2)*k2*(pqd(2)-w(2))+1.0*dq;
taor  = mysatsingle(J(3,3)*k2_scaled*(rd-w(3))+1.0*dr,1.0);

dpqr = [dp; dq; dr];

== matlab function FTC_Unknown/innerloop/dr ==
  data: fd input single size=1; taop input single size=1; taoq input single size=1; taor input single size=1; T output single size=4; B input single size=[4,4]
function T  = fcn(fd, taop, taoq, taor, B)
%% 求解
vd = [fd; taop; taoq; taor];

T1 = B(1,:)*vd;
T2 = B(2,:)*vd;
T3 = B(3,:)*vd;
T4 = B(4,:)*vd;
T = [T1; T2; T3; T4];
% T=min(max(B*vd,[single(0);single(0);single(0);single(0)]),[single(3); single(3); single(3); single(3)]);

== matlab function FTC_Unknown/innerloop/fmincon ==
  data: fd input; taop input; taoq input; taor input; T output; T0 input; M input; val output; time output
function [T,val,time] = fcn(fd, taop, taoq, taor, T0, M)
%% 求解
w1= 1;
w2 =20;
w3= 20;
w4= 0.00;
myfun2 = @(x)(w1*(M(1,:)*x-fd)^2+w2*(M(2,:)*x-taop)^2+w3*(M(3,:)*x-taoq)^2+w4*(M(4,:)*x-taor)^2);

lb  = [0 0 0 0]';
ub  = [3 3 3 3]';

options = optimoptions(@fmincon,'Algorithm','sqp','MaxIterations',10);
% tic
[T,val] = fmincon(myfun2,T0,[],[],[],[],lb,ub,[],options);
% ff = toc;
time =0;

== matlab function FTC_Unknown/innerloop/quadprog ==
  data: fd input double; taop input double; taoq input double; taor input double; T output double; T0 input double; M input double; fval output double; ub input double; iter output
function [T,fval, iter] = fcn(fd, taop, taoq, taor, T0, M, ub)
%% 求解
vd = [fd; taop; taoq; taor];
W=diag([1 20 20 0.01]);
H = M'*W*M;
f = -(vd'*W*M)';
% Td = B*vd;
lb  = [0 0 0 0]';
% ub  = [12 12 12 12]';
% if (max(B*vd)>3)||(min(B*vd)<0)
    options = optimoptions(@quadprog,'Algorithm','active-set','MaxIterations',10);

    [T,fval,~,output] = quadprog(H, f, [], [], [], [], lb, ub, T0, options);
     iter = output.iterations;
% else
%     T = B*vd;
%     fval = 0;
% end

== matlab function FTC_Unknown/innerloop/MATLAB Function1 ==
  data: u input; y output
function y = fcn(u)
y=diag([u,1,1,1]);

== matlab function FTC_Unknown/innerloop/MATLAB Function2 ==
  data: dT input; ub output
function ub = fcn(dT)
dub = zeros(4,1);
dub(1) = dT(1) - dT(3);
dub(2) = dT(2) - dT(4);
dub(3) = dT(3) - dT(1);
dub(4) = dT(4) - dT(2);
% dub(1) = dT(1);
% dub(2) = dT(2);
% dub(3) = dT(3);
% dub(4) = dT(4);
ub = [5 5 5 5]' + 1.8*min([dub(1) dub(2) dub(3) dub(4)]',[0 0 0 0]');%1.8

== matlab function FTC_Unknown/InputConditioning/MATLAB Function ==
  data: u input; y output
function y = fcn(u)

 if(u>1550)
    y=u;
 else
     if(u<1450)
     y=u;
     else
         y=single(1500);
     end
 end

== matlab function FTC_Unknown/InputConditioning/MATLAB Function1 ==
  data: u input; y output
function y = fcn(u)

 if(u>1550)
    y=u;
 else
     if(u<1450)
     y=u;
     else
         y=single(1500);
     end
 end

== matlab function FTC_Unknown/InputConditioning/MATLAB Function2 ==
  data: u input; y output
function y = fcn(u)

 if(u>1550)
    y=u;
 else
     if(u<1450)
     y=u;
     else
         y=single(1500);
     end
 end

== matlab function FTC_Unknown/quat2eul ==
  data: q input single; dcm output single
function dcm  = quat2eul(q)
% Conversion from Quaternion to Euler angles based on the PX4 Firmware
% v1.6.5 release.
% 
% Quaternion -> DCM -> Euler Angles
% INPUT:
%   q: Quaternion vector of the format: (a + bi + cj + dk)
% OUTPUT:
%   [phi,theta,psi]: Euler angles in radians.
% 
 if norm(q)~=0
    a = q(1);
    b = q(2);
    c = q(3);
    d = q(4);

    aSq = a*a;
    bSq = b*b;
    cSq = c*c;
    dSq = d*d;

    d_pi2 = pi/2;

    % quaternion_to_dcm
    dcm00 = aSq + bSq - cSq - dSq;
    dcm01 = 2*(b*c - a*d);
    dcm02 = 2*(a*c + b*d);
    dcm10 = 2*(b*c + a*d);
    dcm11 = aSq - bSq + cSq - dSq;
    dcm12 = 2*(c*d - a*b);
    dcm20 = 2*(b*d - a*c);
    dcm21 = 2*(a*b + c*d);
    dcm22 = aSq - bSq - cSq + dSq;
    dcm=[dcm00 dcm01 dcm02;
              dcm10 dcm11 dcm12;
              dcm20 dcm21  dcm22];
 else
     dcm = single(eye(3,3));
 end
    % dcm_to_euler

== matlab function FTC_Unknown/innerloop/Att ==
  data: e input; w input; psi input; pqrd output; ATT_P input; ATT_P_SCALE input
function pqrd  = fcn(e, w, psi, ATT_P, ATT_P_SCALE)
%% 角度控制1
% h1 = n3(1);
% h2 = n3(2);
% h3 = n3(3);
% h1d = n3d(1);
% h2d = n3d(2);
% h3d = n3d(3);
% we = Reb*w;
% k1 = single(5);
% epqd = [0 -1/h3; 1/h3 0]*[k1*(h1d-h1)+h2*we(3);k1*(h2d-h2)-h1*we(3)];
% 
% psid = single(0);
% rd = k1*0.3*(psid - psi);
% 
% Rbe = Reb';
% erd = (rd - Rbe(3,1)*epqd(1) - Rbe(3,2)*epqd(2))/Rbe(3,3);
% 
% pqd = Rbe((1:2),:)*[epqd; erd];%计算出机体系下的pqd
% pqd = mysat(pqd,2);
% pqrd = [pqd;rd];
%% 角度控制2
e1 = e(1);
e2 = e(2);
% e1  = n3(1) - n3d(1);
% e2  = n3(2) - n3d(2); 
beta = atan2(e2,e1);

k1 = ATT_P;
pqd = [ -k1*sqrt(e1^2+e2^2)*sin(psi-beta);
             -k1*sqrt(e1^2+e2^2)*cos(psi-beta);];
pqd = mysatsingle(pqd,3);
psid = 0;
% rd = -k1*0.3*(psi-psid);
rd = -k1*ATT_P_SCALE*(psi-psid);
% rd = 0;
pqrd = [pqd;rd];

== matlab function FTC_Unknown/Subsystem1/d_z ==
  data: n3 input size=[3,1]; dvz input single size=1; T_ input single size=4; M input single size=[4,4]; m input single size=1; g input single size=1; dz output single size=1
function dz   = fcn(n3, dvz, T_, M, m, g)
dz  = m*(dvz-g)/n3(3)+M(1,:)*T_;

== matlab function FTC_Unknown/Subsystem1/MATLAB Function2 ==
  data: throtte input; ad output; p input; v input; vhd input; POS_P input; VEL_P input
function ad = fcn(throtte, p, v, vhd, POS_P, VEL_P)
persistent pd
if isempty(pd)
    pd = single(p);
end
%% 高度通道
if throtte>=0.4&& throtte <=0.6
        vd3 = mysatsingle(POS_P * (pd(3) - p(3)), 0.5);
        ad3 = VEL_P * (vd3 - v(3));
else
    if throtte>0.6
        vd3 = -1;
        ad3 = VEL_P * (vd3 - v(3));
        pd(3) = p(3);
    else
        vd3 = 1;
        ad3 = VEL_P * (vd3 - v(3));
        pd(3) = p(3);
    end
end
%% 水平通道
if norm(vhd) <= 0.05
        vd12 = mysatsingle(POS_P * (pd(1:2) - p(1:2)), 0.5);
        ad12 = VEL_P * (vd12 - v(1:2));
else
        vd12 = mysatsingle(5*vhd, 0.7);%0.7
        ad12 = VEL_P * (vd12 - v(1:2));
        pd(1:2) = p(1:2);
end
ad = [ad12;ad3];

== matlab function FTC_Unknown/Subsystem2/MATLAB Function ==
  data: Reb input; psi output
function psi = fcn(Reb)
psi = atan2(Reb(2,1), Reb(1,1));

== matlab function FTC_Unknown/Subsystem1/Pos ==
  data: ad3 input single size=[3,1]; n3 input; m input single size=1; fd output single size=1; g input single size=1; n3d output single size=3; ad output single size=3; SAT_AD input
function [fd, n3d, ad]  = fcn(ad3, n3, m, g, SAT_AD)
 

% ad3 = [ad1(1)+ad2(1); ad1(2)+ad2(2); ad1(3)+ad2(3)];

ad = mysatsingle(ad3,single(SAT_AD)*g);

n3d = ([single(0); single(0); g]-ad)/norm([single(0); single(0); g]-ad);
if n3d(3)==single(0)
    fd = single(0);
else
    fd = m*(g-ad(3))/n3(3);
%     fd = m*g-ad(3);
end
